simulink model "Synchronous_2017"  (R2017a)
settings: Solver=VariableStepAuto  StartTime=0.0  StopTime=0.1  MaxStep=1e-4  MinStep=1e-5  RelTol=1e-3
values from neighbouring files (symbols this model uses):
  B = 11e-5    (= 0.00011)    [parameters.m]
  J = 0.47e-4    (= 4.7e-05)    [parameters.m]
  Ld = 0.0031    [parameters.m]
  Lq = 0.004    [parameters.m]
  p = 2    [parameters.m]
  Rs = 2.98    [parameters.m]
libraries: powerlib_meascontrol x1
settings Model: Creator=Omid  LastModifiedBy=Omid
settings DataIOCC: ReturnWorkspaceOutputs=on
settings DebuggingCC: UnconnectedInputMsg=none  UnconnectedOutputMsg=none  UnconnectedLineMsg=none
settings ModelReferenceCC: EnableRefExpFcnMdlSchedulingChecks=off
settings SFSimCC: SimUseLocalCustomCode=on
settings RTWCC: RTWUseLocalCustomCode=on

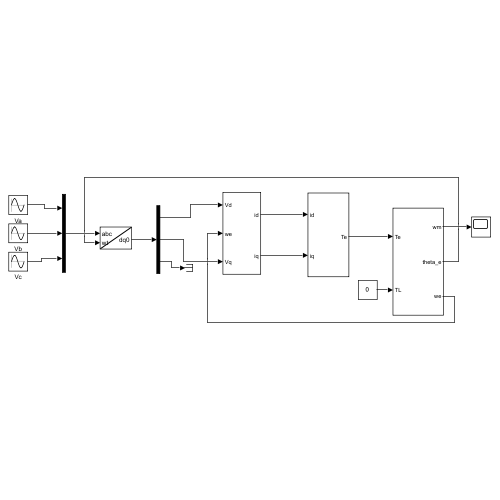
[thumbnail: Simulink's stored preview of the top-level diagram]
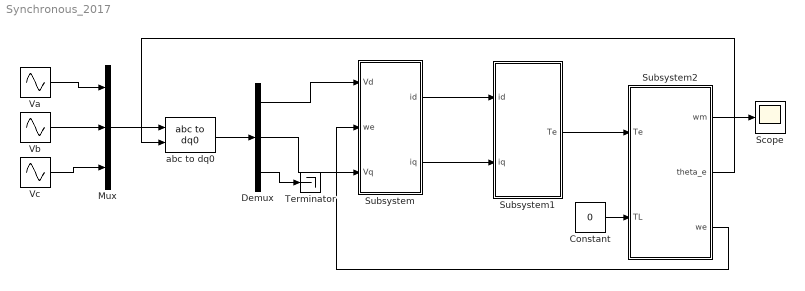
== system Synchronous_2017 ==
  Constant : Constant  Value=0
  Demux : Demux  Outputs=3
  Mux : Mux  Inputs=3
  Scope : Scope
  Subsystem : Subsystem
  Subsystem1 : Subsystem
  Subsystem2 : Subsystem
  Terminator : Terminator
  Va : Sin  Amplitude=240  Frequency=2*pi*50  SampleTime=0
  Vb : Sin  Amplitude=240  Frequency=2*pi*50  Phase=-2*pi/3  SampleTime=0
  Vc : Sin  Amplitude=240  Frequency=2*pi*50  Phase=2*pi/3  SampleTime=0
  abc to dq0 : powerlib_meascontrol/Transformations/abc to dq0  Alignment=Aligned with phase A axis
  wires:
  Subsystem/1(id) -> Subsystem1/1(id)
  Subsystem/2(iq) -> Subsystem1/2(iq)
  Subsystem1/1(Te) -> Subsystem2/1(Te)
  Subsystem2/3(we) -> Subsystem/2(we)
  Va/1 -> Mux/1
  Vb/1 -> Mux/2
  Vc/1 -> Mux/3
  Mux/1 -> abc to dq0/1
  abc to dq0/1 -> Demux/1
  Demux/1 -> Subsystem/1(Vd)
  Subsystem2/2(theta_e) -> abc to dq0/2
  Demux/2 -> Subsystem/3(Vq)
  Demux/3 -> Terminator/1
  Constant/1 -> Subsystem2/2(TL)
  Subsystem2/1(wm) -> Scope/1

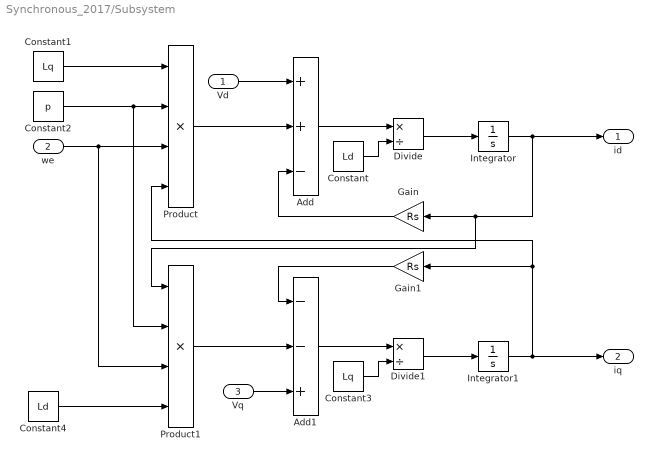
== system Synchronous_2017/Subsystem ==
  Vd : Inport
  we : Inport  Port=2
  Vq : Inport  Port=3
  Add : Sum  Inputs=++-
  Add1 : Sum  Inputs=--+
  Constant : Constant  Value=Ld
  Constant1 : Constant  Value=Lq
  Constant2 : Constant  Value=p
  Constant3 : Constant  Value=Lq
  Constant4 : Constant  Value=Ld
  Divide : Product  Inputs=*/
  Divide1 : Product  Inputs=*/
  Gain : Gain  Gain=Rs
  Gain1 : Gain  Gain=Rs
  Integrator : Integrator
  Integrator1 : Integrator
  Product : Product  Inputs=4
  Product1 : Product  Inputs=4
  id : Outport
  iq : Outport  Port=2
  wires:
  Vq/1 -> Add1/3
  Integrator/1 -> id/1, Product1/1, Gain/1
  Gain1/1 -> Add1/1
  Constant1/1 -> Product/1
  Gain/1 -> Add/3
  Product/1 -> Add/2
  Product1/1 -> Add1/2
  Add/1 -> Divide/1
  Constant2/1 -> Product1/2, Product/2
  Constant4/1 -> Product1/4
  Integrator1/1 -> iq/1, Product/4, Gain1/1
  Vd/1 -> Add/1
  Divide/1 -> Integrator/1
  Constant/1 -> Divide/2
  Constant3/1 -> Divide1/2
  Add1/1 -> Divide1/1
  we/1 -> Product1/3, Product/3
  Divide1/1 -> Integrator1/1

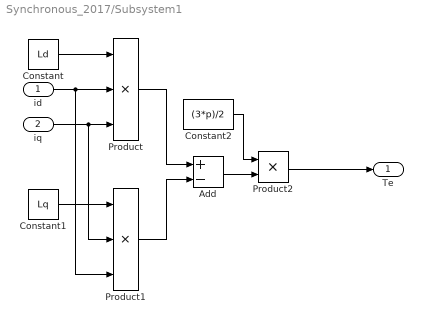
== system Synchronous_2017/Subsystem1 ==
  id : Inport
  iq : Inport  Port=2
  Add : Sum  Inputs=+-
  Constant : Constant  Value=Ld
  Constant1 : Constant  Value=Lq
  Constant2 : Constant  Value=(3*p)/2
  Product : Product  Inputs=3
  Product1 : Product  Inputs=3
  Product2 : Product
  Te : Outport
  wires:
  Product2/1 -> Te/1
  id/1 -> Product1/3, Product/2
  iq/1 -> Product1/2, Product/3
  Product1/1 -> Add/2
  Product/1 -> Add/1
  Constant1/1 -> Product1/1
  Constant/1 -> Product/1
  Add/1 -> Product2/2
  Constant2/1 -> Product2/1

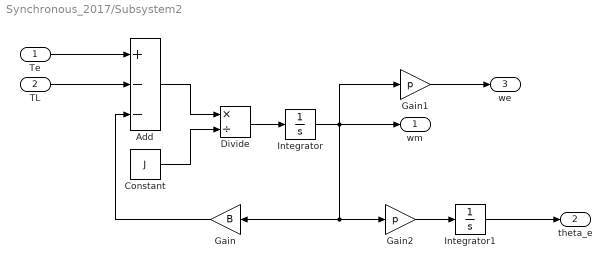
== system Synchronous_2017/Subsystem2 ==
  Te : Inport
  TL : Inport  Port=2
  Add : Sum  Inputs=+--
  Constant : Constant  Value=J
  Divide : Product  Inputs=*/
  Gain : Gain  Gain=B
  Gain1 : Gain  Gain=p
  Gain2 : Gain  Gain=p
  Integrator : Integrator
  Integrator1 : Integrator
  wm : Outport
  theta_e : Outport  Port=2
  we : Outport  Port=3
  wires:
  Constant/1 -> Divide/2
  Integrator/1 -> wm/1, Gain2/1, Gain/1, Gain1/1
  Gain1/1 -> we/1
  Gain2/1 -> Integrator1/1
  Integrator1/1 -> theta_e/1
  Gain/1 -> Add/3
  Divide/1 -> Integrator/1
  TL/1 -> Add/2
  Te/1 -> Add/1
  Add/1 -> Divide/1
